simulink model "sgMdl_BMTS_TemperatureSensorEmulationWithTSE"  (R2024b)
settings: Solver=FixedStepAuto  StartTime=0.0  StopTime=inf  RelTol=1e-3  EnableMultiTasking=on
undefined symbols (not defined in the file): Device_01, sg_bce, TSE04, TSE_4Ch_Set_init, TSE_Ch1, TSE_Ch2, TSE_Ch3, TSE_Ch4
libraries: slrealtimeethercatlib x11, simulink x1, SignalEditorBlockLib x1
Description:
  | BMTS - Temperature Sensor Emulation with TSE
settings Model: ModifiedByFormat=Speedgoat  SimulationMode=external  ExtModeTrigDuration=100000  Creator=Speedgoat  LastModifiedBy=Speedgoat
settings SolverCC: ConcurrentTasks=on  AlgebraicLoopSolver=TrustRegion  PositivePriorityOrder=on  InsertRTBMode=Never (minimum delay)
settings DataIOCC: SaveFormat=Array  SaveState=on  SignalLoggingName=logsOut
settings OptimizationCC: BlockReduction=off  BooleanDataType=off  OptimizeBlockIOStorage=off  BufferReuse=off  ReuseModelBlockBuffer=off  GlobalBufferReuse=off  ExpressionFolding=off  LocalBlockOutputs=off  InitFltsAndDblsToZero=on  OptimizeDataStoreBuffers=off  BusAssignmentInplaceUpdate=off
settings DebuggingCC: SaveWithParameterizedLinksMsg=none  MergeDetectMultiDrivingBlocksExec=none  CheckExecutionContextPreStartOutputMsg=on  SignalResolutionControl=TryResolveAllWithWarning  TasksWithSamePriorityMsg=none  UnconnectedInputMsg=warning  UnconnectedOutputMsg=warning  UnconnectedLineMsg=warning  SFUnexpectedBacktrackingDiag=warning  SFNoUnconditionalDefaultTransitionDiag=warning  SFExecutionAtInitializationDiag=none  ArithmeticOperatorsInVariantConditions=warning
settings HardwareCC: ProdBitPerLong=64  ProdLongLongMode=on  ProdHWDeviceType=Intel->x86-64 (Linux 64)
settings ModelReferenceCC: EnableRefExpFcnMdlSchedulingChecks=on  PropagateSignalLabelsOutOfModel=off
settings SFSimCC: SimUseLocalCustomCode=off  SimTargetLang=C++
settings RTWCC: Description=Speedgoat Real-Time Target Machine  SystemTargetFile=speedgoat.tlc  TemplateMakefile=slrealtime_default_tmf  RTWUseLocalCustomCode=off  Toolchain=Simulink Real-Time Toolchain  BuildConfiguration=Faster Runs  TargetLang=C++  GPUComputeCapability=3.5  DLArmComputeVersion=19.05
settings CodeAppCC: StateflowObjectComments=on
settings SimulinkRealTimeTargetCC: SubcomponentCodeInterfacePackaging=Reusable function  InstructionSetFMA=off  LogToMDFFile=off  SLRTFileLogMaxRuns=10
settings ConfigComp: CovMetricSettings=dw  CovSaveCumulativeToWorkspaceVar=on  CovSaveSingleToWorkspaceVar=on  CovExternalEMLEnable=off  CovSFcnEnable=off  CovBoundaryAbsTol=1.0e-5

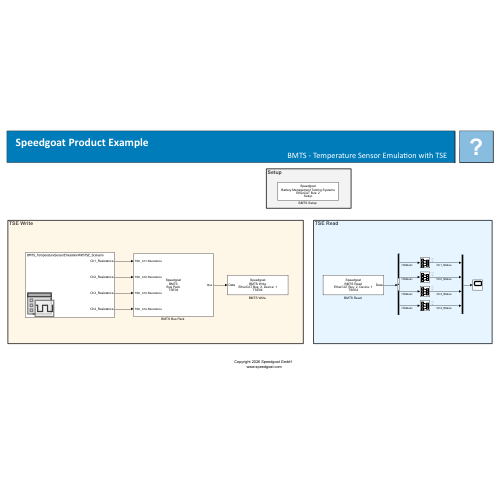
[thumbnail: Simulink's stored preview of the top-level diagram]
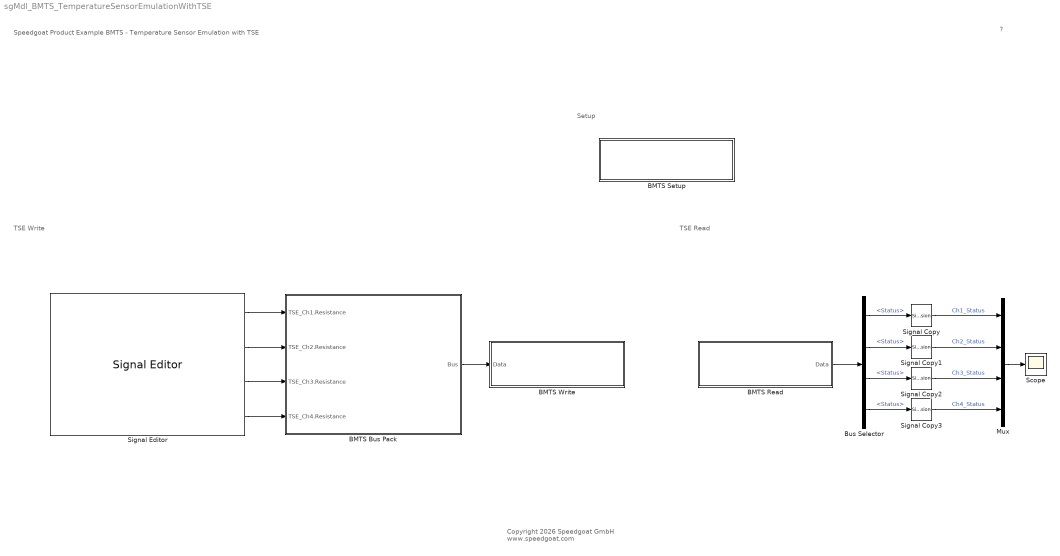
== system sgMdl_BMTS_TemperatureSensorEmulationWithTSE ==
  note: Setup
  note: TSE Write
  note: TSE Read
  note: Speedgoat Product Example
      | BMTS - Temperature Sensor Emulation with TSE
  note: ?
  note: Copyright 2026 Speedgoat GmbH
      |  www.speedgoat.com
  "BMTS Bus Pack " : Subsystem  mask(bmts_bus_pack){}
      settings: OpenFcn=sg_bce.openFcnBuspack;
      mask Help: eval('sg.utils.help.show(''io_main/refentry_bmts_buspack'');')
      mask Display: disp('Speedgoat\nBMTS\nBus Pack\nTSE04');
  "BMTS Read " : Subsystem  LoadFcn=sg_bce.createFiuTseBusSignals(0,4);  InitFcn=|  mask(bce_read){}
      | sg_bce.createFiuTseBusSignals(0,4);
      | sg_bce.checkNumberOfBlocksGlobal(bdroot);
      settings: OpenFcn=sg_bce.openFcnRead;
      mask Help: eval('sg.utils.help.show(''io_main/refentry_bce_read'');')
      mask Display: disp('Speedgoat\nBMTS Read\nEtherCAT Bus: 2, Device: 1\nTSE04');port_label('output',1,'Data');
  "BMTS Setup " : Subsystem  LoadFcn=|  InitFcn=|  mask(bce_setup){}
      LoadFcn=|
      | sg_bce.createBusSignals;
      | sg_bce.setupEniCallback(gcb, bdroot);
      InitFcn=|
      | sg_bce.createBusSignals;
      | sg_bce.checkNumberOfBlocksGlobal(bdroot);
      | sg_bce.setupEniCallback(gcb, bdroot);
      settings: OpenFcn=sg_bce.openFcnSetup;
      mask Help: eval('sg.utils.help.show(''io_main/refentry_bce_setup'');')
      mask Display: disp('Speedgoat\nBattery Management Testing Systems\nEtherCAT Bus: 2\nSetup');
  "BMTS Write " : Subsystem  LoadFcn=sg_bce.createFiuTseBusSignals(0,4);  InitFcn=|  mask(bce_write){}
      | sg_bce.createFiuTseBusSignals(0,4);
      | sg_bce.checkNumberOfBlocksGlobal(bdroot);
      settings: OpenFcn=sg_bce.openFcnWrite;
      mask Help: eval('sg.utils.help.show(''io_main/refentry_bce_write'');')
      mask Display: disp('Speedgoat\nBMTS Write\nEtherCAT Bus: 2, Device: 1\nTSE04');port_label('input',1,'Data');
  Bus Selector : BusSelector  OutputSignals=TSE_Ch1.Status,TSE_Ch2.Status,TSE_Ch3.Status,TSE_Ch4.Status
  Mux : Mux
  Scope : Scope
  Signal Copy{,1..3} (4 alike) : SignalConversion  OverrideOpt=off
  Signal Editor : SignalEditorBlockLib/Signal Editor  FileName=BMTS_TemperatureSensorEmulationWithTSE_Scenario.mat  ActiveScenario=BMTS_TemperatureSensorEmulationWithTSE_Scenario  ActiveSignal=Ch1_Resistance  IsBus=off  OutputBusObjectStr=Bus: BusObject  SampleTime=0  Interpolate=off  ZeroCross=off  OutputAfterFinalValue=Holding final value  Unit=inherit  PreserveSignalName=on  ApplySigPropsToAllScenarios=on  ApplySigPropsToAllSignals=off
  wires:
  "BMTS Bus Pack "/1(Bus) -> "BMTS Write "/1(Data)
  "BMTS Read "/1(Data) -> Bus Selector/1
  Bus Selector/1 -> Signal Copy/1  "<Status>"
  Bus Selector/2 -> Signal Copy1/1  "<Status>"
  Bus Selector/3 -> Signal Copy2/1  "<Status>"
  Bus Selector/4 -> Signal Copy3/1  "<Status>"
  Mux/1 -> Scope/1
  Signal Editor/1 -> "BMTS Bus Pack "/1(TSE_Ch1.Resistance)
  Signal Editor/2 -> "BMTS Bus Pack "/2(TSE_Ch2.Resistance)
  Signal Editor/3 -> "BMTS Bus Pack "/3(TSE_Ch3.Resistance)
  Signal Editor/4 -> "BMTS Bus Pack "/4(TSE_Ch4.Resistance)
  Signal Copy/1 -> Mux/1  "Ch1_Status"
  Signal Copy1/1 -> Mux/2  "Ch2_Status"
  Signal Copy2/1 -> Mux/3  "Ch3_Status"
  Signal Copy3/1 -> Mux/4  "Ch4_Status"

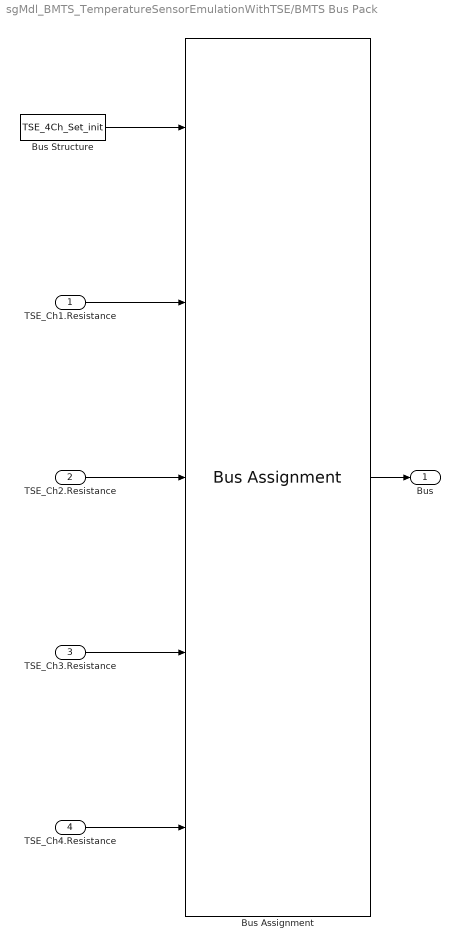
== system sgMdl_BMTS_TemperatureSensorEmulationWithTSE/BMTS Bus Pack  ==
  TSE_Ch1.Resistance : Inport
  TSE_Ch2.Resistance : Inport  Port=2
  TSE_Ch3.Resistance : Inport  Port=3
  TSE_Ch4.Resistance : Inport  Port=4
  Bus Assignment : BusAssignment  AssignedSignals=TSE_Ch1.Resistance,TSE_Ch2.Resistance,TSE_Ch3.Resistance,TSE_Ch4.Resistance
  Bus Structure : Constant  Value=TSE_4Ch_Set_init  OutDataTypeStr=Bus: TSE_4Ch_Set
  Bus : Outport
  wires:
  Bus Structure/1 -> Bus Assignment/1
  Bus Assignment/1 -> Bus/1
  TSE_Ch2.Resistance/1 -> Bus Assignment/3
  TSE_Ch1.Resistance/1 -> Bus Assignment/2
  TSE_Ch3.Resistance/1 -> Bus Assignment/4
  TSE_Ch4.Resistance/1 -> Bus Assignment/5

== system sgMdl_BMTS_TemperatureSensorEmulationWithTSE/BMTS Read  ==
  Subsystem : Subsystem
  Data : Outport  OutDataTypeStr=Bus: TSE_4Ch_Get
  wires:
  Subsystem/1(Data) -> Data/1

== system sgMdl_BMTS_TemperatureSensorEmulationWithTSE/BMTS Setup  ==
  EtherCAT Init : slrealtimeethercatlib/EtherCAT Init  Priority=0  config_file=C:\Users\timo.straessle\AppData\Local\Temp\sg_bmts\sgMdl_BMTS_TemperatureSensorEmulationWithTSE\sg_bmts_ENI_bus2.xml  device_id=2  portnum=1  initstate=2  dctuning=0  enaDebug=0  logFile='c:\dbglog.txt'  sample_time=0.001000  DCMode=0
  Terminator : Terminator
  wires:
  EtherCAT Init/1 -> Terminator/1

== system sgMdl_BMTS_TemperatureSensorEmulationWithTSE/BMTS Write  ==
  Data : Inport  OutDataTypeStr=Bus: TSE_4Ch_Set
  Subsystem : Subsystem
  wires:
  Data/1 -> Subsystem/1(Data)

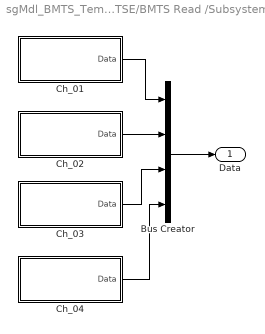
== system sgMdl_BMTS_TemperatureSensorEmulationWithTSE/BMTS Read /Subsystem ==
  Bus Creator : BusCreator  Inputs=4  OutDataTypeStr=Bus: TSE_4Ch_Get
      settings: InheritFromInputs=off
  Ch_01 : Subsystem
  Ch_02 : Subsystem
  Ch_03 : Subsystem
  Ch_04 : Subsystem
  Data : Outport  OutDataTypeStr=Bus: TSE_4Ch_Get
  wires:
  Ch_01/1(Data) -> Bus Creator/1
  Ch_02/1(Data) -> Bus Creator/2
  Bus Creator/1 -> Data/1
  Ch_04/1(Data) -> Bus Creator/4
  Ch_03/1(Data) -> Bus Creator/3

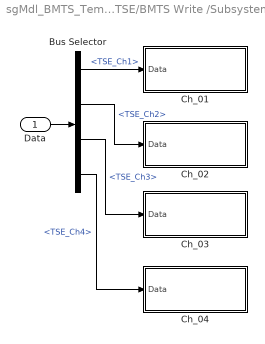
== system sgMdl_BMTS_TemperatureSensorEmulationWithTSE/BMTS Write /Subsystem ==
  Data : Inport  OutDataTypeStr=Bus: TSE_4Ch_Set
  Bus Selector : BusSelector  OutputSignals=TSE_Ch1,TSE_Ch2,TSE_Ch3,TSE_Ch4
  Ch_01 : Subsystem
  Ch_02 : Subsystem
  Ch_03 : Subsystem
  Ch_04 : Subsystem
  wires:
  Bus Selector/2 -> Ch_02/1(Data)  "<TSE_Ch2>"
  Bus Selector/1 -> Ch_01/1(Data)  "<TSE_Ch1>"
  Data/1 -> Bus Selector/1
  Bus Selector/4 -> Ch_04/1(Data)  "<TSE_Ch4>"
  Bus Selector/3 -> Ch_03/1(Data)  "<TSE_Ch3>"

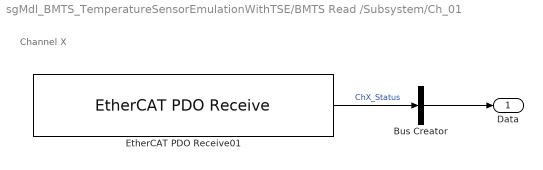
== system sgMdl_BMTS_TemperatureSensorEmulationWithTSE/BMTS Read /Subsystem/Ch_01 ==
  note: Channel X
  Bus Creator : BusCreator  Inputs=1  OutDataTypeStr=Bus: TSE_Get
      settings: InheritFromInputs=off
  EtherCAT PDO Receive01 : slrealtimeethercatlib/EtherCAT PDO Receive  Priority=2  sig_name=Device_01 (TSE04).Tx_Channel_01.status  sig_offset=0  sig_type=single  type_size=32  sig_dim=1  device_id=2  sample_time=0.001000
  Data : Outport  OutDataTypeStr=Bus: TSE_Get
  wires:
  Bus Creator/1 -> Data/1
  EtherCAT PDO Receive01/1 -> Bus Creator/1  "ChX_Status"

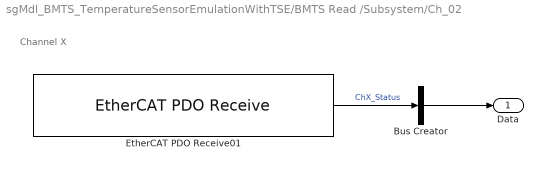
== system sgMdl_BMTS_TemperatureSensorEmulationWithTSE/BMTS Read /Subsystem/Ch_02 ==
  note: Channel X
  Bus Creator : BusCreator  Inputs=1  OutDataTypeStr=Bus: TSE_Get
      settings: InheritFromInputs=off
  EtherCAT PDO Receive01 : slrealtimeethercatlib/EtherCAT PDO Receive  Priority=2  sig_name=Device_01 (TSE04).Tx_Channel_02.status  sig_offset=32  sig_type=single  type_size=32  sig_dim=1  device_id=2  sample_time=0.001000
  Data : Outport  OutDataTypeStr=Bus: TSE_Get
  wires:
  Bus Creator/1 -> Data/1
  EtherCAT PDO Receive01/1 -> Bus Creator/1  "ChX_Status"

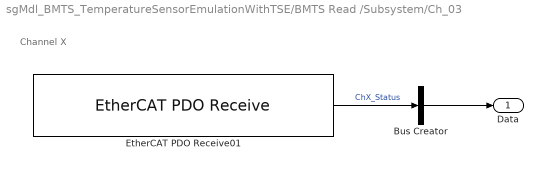
== system sgMdl_BMTS_TemperatureSensorEmulationWithTSE/BMTS Read /Subsystem/Ch_03 ==
  note: Channel X
  Bus Creator : BusCreator  Inputs=1  OutDataTypeStr=Bus: TSE_Get
      settings: InheritFromInputs=off
  EtherCAT PDO Receive01 : slrealtimeethercatlib/EtherCAT PDO Receive  Priority=2  sig_name=Device_01 (TSE04).Tx_Channel_03.status  sig_offset=64  sig_type=single  type_size=32  sig_dim=1  device_id=2  sample_time=0.001000
  Data : Outport  OutDataTypeStr=Bus: TSE_Get
  wires:
  Bus Creator/1 -> Data/1
  EtherCAT PDO Receive01/1 -> Bus Creator/1  "ChX_Status"

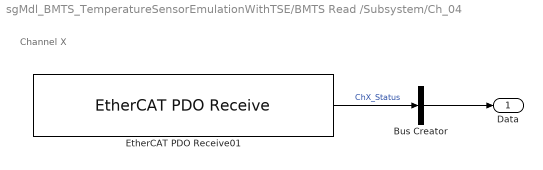
== system sgMdl_BMTS_TemperatureSensorEmulationWithTSE/BMTS Read /Subsystem/Ch_04 ==
  note: Channel X
  Bus Creator : BusCreator  Inputs=1  OutDataTypeStr=Bus: TSE_Get
      settings: InheritFromInputs=off
  EtherCAT PDO Receive01 : slrealtimeethercatlib/EtherCAT PDO Receive  Priority=2  sig_name=Device_01 (TSE04).Tx_Channel_04.status  sig_offset=96  sig_type=single  type_size=32  sig_dim=1  device_id=2  sample_time=0.001000
  Data : Outport  OutDataTypeStr=Bus: TSE_Get
  wires:
  Bus Creator/1 -> Data/1
  EtherCAT PDO Receive01/1 -> Bus Creator/1  "ChX_Status"

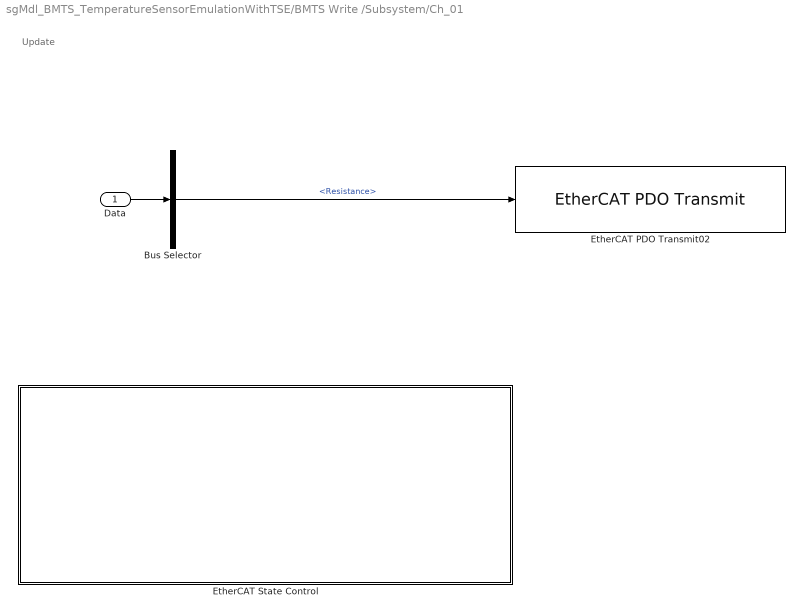
== system sgMdl_BMTS_TemperatureSensorEmulationWithTSE/BMTS Write /Subsystem/Ch_01 ==
  note: Update
  Data : Inport  OutDataTypeStr=Bus: TSE_Set
  Bus Selector : BusSelector  OutputSignals=Resistance
  EtherCAT PDO Transmit02 : slrealtimeethercatlib/EtherCAT PDO Transmit  Priority=3  sig_name=Device_01 (TSE04).Rx_Channel_01.resistance  sig_offset=0  sig_type=double  type_size=64  sig_dim=1  device_id=2  sample_time=0.001000
  EtherCAT State Control : Subsystem
  wires:
  Bus Selector/1 -> EtherCAT PDO Transmit02/1  "<Resistance>"
  Data/1 -> Bus Selector/1

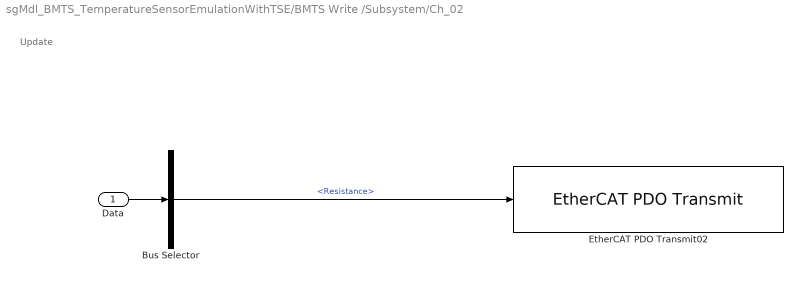
== system sgMdl_BMTS_TemperatureSensorEmulationWithTSE/BMTS Write /Subsystem/Ch_02 ==
  note: Update
  Data : Inport  OutDataTypeStr=Bus: TSE_Set
  Bus Selector : BusSelector  OutputSignals=Resistance
  EtherCAT PDO Transmit02 : slrealtimeethercatlib/EtherCAT PDO Transmit  Priority=3  sig_name=Device_01 (TSE04).Rx_Channel_02.resistance  sig_offset=64  sig_type=double  type_size=64  sig_dim=1  device_id=2  sample_time=0.001000
  wires:
  Bus Selector/1 -> EtherCAT PDO Transmit02/1  "<Resistance>"
  Data/1 -> Bus Selector/1

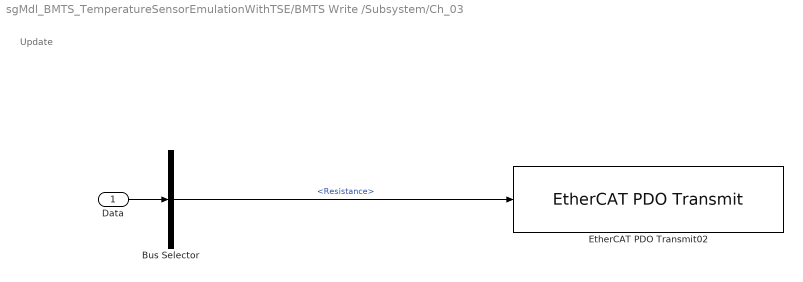
== system sgMdl_BMTS_TemperatureSensorEmulationWithTSE/BMTS Write /Subsystem/Ch_03 ==
  note: Update
  Data : Inport  OutDataTypeStr=Bus: TSE_Set
  Bus Selector : BusSelector  OutputSignals=Resistance
  EtherCAT PDO Transmit02 : slrealtimeethercatlib/EtherCAT PDO Transmit  Priority=3  sig_name=Device_01 (TSE04).Rx_Channel_03.resistance  sig_offset=128  sig_type=double  type_size=64  sig_dim=1  device_id=2  sample_time=0.001000
  wires:
  Bus Selector/1 -> EtherCAT PDO Transmit02/1  "<Resistance>"
  Data/1 -> Bus Selector/1

== system sgMdl_BMTS_TemperatureSensorEmulationWithTSE/BMTS Write /Subsystem/Ch_04 ==
  note: Update
  Data : Inport  OutDataTypeStr=Bus: TSE_Set
  Bus Selector : BusSelector  OutputSignals=Resistance
  EtherCAT PDO Transmit02 : slrealtimeethercatlib/EtherCAT PDO Transmit  Priority=3  sig_name=Device_01 (TSE04).Rx_Channel_04.resistance  sig_offset=192  sig_type=double  type_size=64  sig_dim=1  device_id=2  sample_time=0.001000
  wires:
  Bus Selector/1 -> EtherCAT PDO Transmit02/1  "<Resistance>"
  Data/1 -> Bus Selector/1

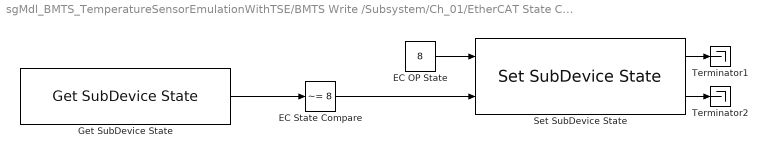
== system sgMdl_BMTS_TemperatureSensorEmulationWithTSE/BMTS Write /Subsystem/Ch_01/EtherCAT State Control ==
  EC OP State : Constant  Value=8  OutDataTypeStr=int32
  EC State Compare : simulink/Logic and Bit Operations/Compare To Constant  relop=~=  const=8  OutDataTypeStr=boolean
  Get SubDevice State : slrealtimeethercatlib/Get SubDevice State  device_id=2  subdevice_name=Device_01 (TSE04)  sample_time=0.001  subdevice_addr=1001  selected_subdevice=Term 1 (EK1100)  timeout=500  subdevice_found=1
  Set SubDevice State : slrealtimeethercatlib/Set SubDevice State  device_id=2  subdevice_name=Device_01 (TSE04)  sample_time=0.001  subdevice_addr=1001  selected_subdevice=Term 1 (EK1100)  subdevice_found=1
  Terminator1 : Terminator
  Terminator2 : Terminator
  wires:
  Set SubDevice State/2 -> Terminator2/1
  EC State Compare/1 -> Set SubDevice State/2
  Set SubDevice State/1 -> Terminator1/1
  Get SubDevice State/1 -> EC State Compare/1
  EC OP State/1 -> Set SubDevice State/1
